simulink model "linear_control_schemes"  (R2019b)
settings: Solver=VariableStepAuto  StartTime=0.0  StopTime=10.0  RelTol=1e-3
settings Model: Creator=Administrator  LastModifiedBy=Administrator

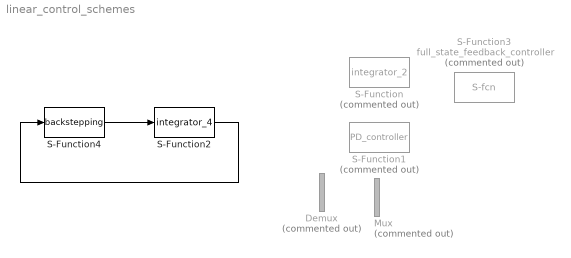
== system linear_control_schemes ==
  Demux : Demux  Commented=on
  Mux : Mux  Commented=on  Inputs=2
  S-Function : S-Function  Commented=on  FunctionName=integrator_2  SFunctionDeploymentMode=off  EnableBusSupport=off
  S-Function1 : S-Function  Commented=on  FunctionName=PD_controller  SFunctionDeploymentMode=off  EnableBusSupport=off
  S-Function2 : S-Function  FunctionName=integrator_4  SFunctionDeploymentMode=off  EnableBusSupport=off
  S-Function3 : S-Function  Commented=on  FunctionName=full_state_feedback_controller  SFunctionDeploymentMode=off  EnableBusSupport=off
  S-Function4 : S-Function  FunctionName=backstepping  SFunctionDeploymentMode=off  EnableBusSupport=off
  wires:
  S-Function4/1 -> S-Function2/1
  S-Function2/1 -> S-Function4/1
